simulink library "Library_SII"  (R2014b)
settings: Solver=ode45  StartTime=0.0  StopTime=10.0  RelTol=1e-3
libraries: fl_lib x77, Library_SII x44, nesl_utility x33, powerlib x15, mblibv1 x11, simulink x6, elec_lib x5, powerlib_extras x1
(part 1 of 4)
settings Model: Creator=Cedrick  LastModifiedBy=Cedrick

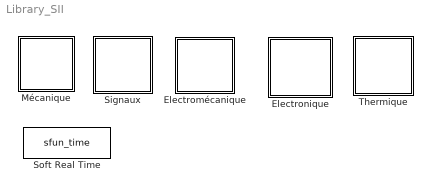
== system Library_SII ==
  Electromécanique : Subsystem
      mask Display: image(imread('Electromecanique.bmp'))
  Electronique : Subsystem
      mask Display: image(imread('Electronique.bmp'))
  Mécanique : Subsystem  mask(Mecanique){}
      mask Display: image(imread('Mecanique.bmp'))
  Signaux : Subsystem
      mask Display: image(imread('Signaux.bmp'))
  Soft Real Time : S-Function  FunctionName=sfun_time  Parameters=x  EnableBusSupport=off  mask{x=1}
      mask prompts: x "Time Scaling Factor"
      mask Display:
      | color('red')
      | disp('Soft Real Time')
  Thermique : Subsystem
      mask Display: image(imread('Thermique.bmp'))

== system Library_SII/Electromécanique ==
  Moteur CC (SPS-SM) : Subsystem  Tag=Moteur  Description=Moteur CC  mask(Moteur CC){axe=[1 0 0], R=0.989, L=0.0000718, K=1.39e-3, J=1.06e-6, kv=0.0002953, kc=0}
      mask prompts: axe "Vecteur directeur [x y z]"; R "Resistance (ohm)"; L "Inductance (H)"; K "Constante de vitesse (V/rpm)"; J "Inertie de l'arbre (kg.m^2)"; kv "Coefficient de frottement visqueux (N.m.s)"; kc "Coefficient de frottement sec"
      mask help:
      | Moteur à courant continu à aimants permanents.
      | L'axe du moteur est défini par le "Vecteur directeur"
      | et par la position du CS relié au stator.
      | Les autres paramètres sont fournis par les constructeurs de moteur.
      |
      | Les ports A+ et A- sont des ports physiques SimPowerSystems.
      | Les ports Stator et Rotor sont des ports mécaniques SimMechanics.
      mask Display:
      | image(imread('Motor.png'))
      | port_label('lconn', 1, 'Stator')
      | port_label('rconn', 1, 'Rotor')
      | port_label('lconn', 2, 'A+')
      | port_label('rconn', 2, 'A-')
  Moteur CC (SPS-SS) : Subsystem  Tag=Moteur  Description=Moteur CC  mask(Moteur CC){R=0.989, L=0.0000718, K=1.39e-3, J=1.06e-6, kv=0.0002953, kc=0}
      mask prompts: R "Resistance (ohm)"; L "Inductance (H)"; K "Constante de vitesse (V/rpm)"; J "Inertie de l'arbre (kg.m^2)"; kv "Coefficient de frottement visqueux (N.m.s)"; kc "Coefficient de frottement sec"
      mask help:
      | Moteur à courant continu à aimants permanents.
      | Les paramètres sont fournis par les constructeurs de moteur.
      |
      | Les ports A+ et A- sont des ports physiques SimPowerSystems.
      | Les ports Stator et Rotor sont des ports mécaniques SimScape.
      mask Display:
      | image(imread('Motor.png'))
      | port_label('lconn', 1, 'Stator')
      | port_label('rconn', 1, 'Rotor')
      | port_label('lconn', 2, 'A+')
      | port_label('rconn', 2, 'A-')
  Moteur PaP (SPS-SS) : Subsystem  Tag=Moteur  Description=Moteur PaP  mask(Moteur CC){R=0.989, L=0.0000718, K=1.39e-3, J=1.06e-6, kv=0.0002953, kc=0}
      mask prompts: R "Resistance (ohm)"; L "Inductance (H)"; K "Constante de vitesse (V/rpm)"; J "Inertie de l'arbre (kg.m^2)"; kv "Coefficient de frottement visqueux (N.m.s)"; kc "Coefficient de frottement sec"
      mask help:
      | Moteur à courant continu à aimants permanents.
      | Les paramètres sont fournis par les constructeurs de moteur.
      |
      | Les ports A+ et A- sont des ports physiques SimPowerSystems.
      | Les ports Stator et Rotor sont des ports mécaniques SimScape.
      mask Display:
      | image(imread('moteur_pap.jpg'))
      | port_label('lconn', 1, 'Stator')
      | port_label('rconn', 1, 'Rotor')
      | port_label('lconn', 2, 'A+')
      | port_label('rconn', 2, 'A-')
      | port_label('lconn', 3, 'B+')
      | port_label('rconn', 3, 'B-')

== system Library_SII/Electronique ==
  Ampèremètre : Subsystem  mask(Ampèremètre){}
      mask help: Ampèremètre avec un signal de sortie au format Simulink
      mask Display:
      | plot([184.371736831963;184.043550999396;183.062154110669;181.436997554304;179.183732476342;176.324059051243;172.885517497347;168.901222849516;164.409546043246;159.453744381582;154.081544943642;148.344684946756;142.298413488781;136.000959469086;129.512970812418;122.896930396238;116.216554306448;109.536178216657;102.920137800477;96.4321491438092;90.134695124114;84.0884236661391;78.3515636692533;72.979364231313;68.0235625696485;63.5318857633786;59.5475911155478;56.1090495616519;53.2493761365527;50.9961110585907;49.3709545022264;48.3895576134986;48.0613717809319;48.3895576134986;49.3709545022264;50.9961110585907;53.2493761365528;56.109049561652;59.547591115548;63.5318857633788;68.0235625696487;72.9793642313131;78.3515636692534;84.0884236661394;90.1346951241142;96.4321491438093;102.920137800477;109.536178216657;116.216554306448;122.896930396238;129.512970812418;136.000959469086;142.298413488781;148.344684946756;154.081544943642;159.453744381582;164.409546043246;168.901222849516;172.885517497347;176.324059051243;179.183732476342;181.436997554304;183.062154110669;184.043550999396;184.371736831963;184.371736831963], [130.389304831624;123.708928741834;117.092888325653;110.604899668986;104.307445649291;98.2611741913157;92.5243141944298;87.1521147564895;82.1963130948251;77.7046362885552;73.7203416407244;70.2818000868285;67.4221266617293;65.1688615837672;63.5437050274029;62.5623081386751;62.2341223061085;62.5623081386751;63.5437050274029;65.1688615837672;67.4221266617293;70.2818000868285;73.7203416407244;77.7046362885552;82.1963130948251;87.1521147564896;92.5243141944299;98.2611741913158;104.307445649291;110.604899668986;117.092888325653;123.708928741834;130.389304831624;137.069680921414;143.685721337595;150.173709994262;156.471164013958;162.517435471932;168.254295468818;173.626494906759;178.582296568423;183.073973374693;187.058268022524;190.49680957642;193.356483001519;195.609748079481;197.234904635845;198.216301524573;198.54448735714;198.216301524573;197.234904635845;195.609748079481;193.356483001519;190.49680957642;187.058268022524;183.073973374693;178.582296568423;173.626494906759;168.254295468818;162.517435471933;156.471164013958;150.173709994263;143.685721337595;137.069680921415;130.389304831624;130.389304831624])
      | plot([0;240.936758928001;240.936758928001;0;0], [255.109509453177;255.109509453177;0;0;255.109509453177])
      | plot([134.798604995012;113.382004201412], [102.043803781271;158.734805881977])
      | plot([113.696954213083;92.9102534428239], [158.419855870306;102.043803781271])
      | plot([143.617205321789;124.720204621553], [102.043803781271;102.043803781271])
      | plot([101.41390375793;84.406603127718], [102.043803781271;102.043803781271])
      | plot([99.2092536762357;127.554754726589], [119.051104411483;119.051104411483])
      | plot([48.1873517856002;0], [130.389304831624;130.389304831624])
      | plot([184.245756827295;212.591257877648;212.591257877648;240.936758928001], [130.389304831624;130.389304831624;65.194652415812;65.194652415812])
      | ;
      | color('red');
      | port_label('output', 1,'I')
      | port_label('LConn', 1,'+')
      | port_label('RConn', 1,'-')
  Cellule Photovoltaique SPS : Subsystem  mask(Cellule Photovoltaique SPS){Voc=0.6, Isc=5, Tjref=25, alpha=3.4e-4, TXI=3, EG=1.11, Rs=0.01, Rsh=50, Eref=1000, N=1.5}
      mask prompts: Voc "Tension à vide (V)"; Isc "Courant de court circuit (A)"; Tjref "Temperature de référence (°C)"; alpha "Coef de courant en température (°C^-1)"; TXI "Coef d'influence de la T°"; EG "Energie d'activation (eV)"; Rs "Résistance interne (Ohms)"; Rsh "Résistance de shunt (Ohm)"; Eref "Ensoleillement de référence (W/m²)"; N "Facteur de qualité"
      mask help:
      | Modèle d'une cellule photovoltaique.
      | En entrée :
      |   Ta : Température ambiante (°C)
      |   Ir : Irradiation (W/m²)
      |
      | En sortie :
      |   Ports physiques SimPowerSystems
      mask init:
      | % Charge de l'electron
      | q = 1.602e-19; % C
      | % Constante de Boltzmann
      | k = 1.38e-23;
      | % Degrés --> Kelvin
      | Kel = 273.15;
      | 
      | qkT = q/(k*(Tjref+Kel)); % 38.9358 à 25°C
      | 
      | % Courant de saturation de la diode (A)
      | % pour I = 0 (circuit ouvert)
      | I0d = ((Voc+Rs*Isc)/Rsh-Isc)/(exp(qkT*Rs*Isc/N)-exp(qkT*Voc/N));
      | 
      | % Courant de référence (A)
      | % pour U = 0 (court circuit)
      | I0 = Isc*(1+Rs/Rsh)+I0d*(exp(qkT*Rs*Isc/N)-1);
      | 
      | % Coef de tension en température (influe sur Iph)
      | beta = -2.17e-3; % mV/°C
      mask Display:
      | image(imread('cellulePV_poly.jpg'))
      | port_label('input', 1, 'Ta')
      | port_label('input', 2, 'Ir')
      | port_label('rconn', 1, '+')
      | port_label('rconn', 2, '-')
  Cellule Photovoltaique avec capteurs U et I SimElectronics : Subsystem  mask(Cellule Photovoltaique (SimElectronics)){typcell=polycristallin, Icc=4.5, Vco=0.601, Tcell=25, shunt=0, mesure=off, IRef=1000, TRef=25, Qf=1.4}
      mask prompts: typcell "Type"; Icc "Courant de court-circuit (A)"; Vco "Tension de circuit ouvert (V)"; Tcell "Température de cellule (°C)"; shunt "Shunter"; mesure "Mesurer le courant et la tension"; IRef "Irradiance de référence (W/m²)"; TRef "Température de référence (°C)"; Qf "Facteur de qualité"
      mask help:
      | Modèle d'une cellule photovoltaique.
      |  - mesure courant/tension
      |  - possibilité de shunter la cellule (par programmation)
      |
      | En entrée :
      |   Ir : Irradiation (W/m²)
      |
      | Connectique : ports physiques SimElectronics
      |
      | Caractéristiques :
      |     Courant de court-circuit (A)
      |     Tension de circuit ouvert (V)
      |     Température (°C) et irradiance (W/m²) de référence
      |
      | Température
      |     Température de cellule (°C)
      |
      | Il est possible de "tester" cette cellule grâce à l'interface graphique "CellulePV_IHM".
      |
      | Voir aussi la classe "pnl_etat_cellule.m" pour la programmation d'IHM.
      mask TypeOptions typcell: monocristallin | polycristallin | amorphe
      mask Callback typcell:
      | t = get_param(gcb, 'typcell');
      | switch t
      |     case 'monocristallin'
      |         n = '1.4';
      |     case 'polycristallin'
      |         n = '2';
      |     case 'amorphe'
      |         n = '10';
      | end
      | set_param(gcb, 'Qf', n)
      mask Display:
      | t = get_param(gcb, 'typcell');
      | switch t
      |     case 'monocristallin'
      |         image(imread('cellulePV_mono.jpg'))
      |     case 'polycristallin'
      |         image(imread('cellulePV_poly.jpg'))
      |     case 'amorphe'
      |         image(imread('cellulePV_amorphe.jpg'))
      | end
      | 
      | port_label('input', 1, 'Ir')
      | port_label('rconn', 1, '+')
      | port_label('rconn', 2, '-')
      | port_label('output', 1, 'I')
      | port_label('output', 2, 'U')
  Diode : Subsystem  mask(Diode){I0d=1e-6, N=1.5}
      mask prompts: I0d "Courant de saturation (A)"; N "Facteur de qualité"
      mask help:
      | Diode selon le modèle de Shockley :
      | Id = Is*(exp(Vd/(N*Vt))-1)
      |     avec Vt = k*Tj/q
      |
      |     Id : courant traversant la diode
      |     Vd : tension aux bornes de la diode
      |
      |     k : constante de Boltzmann
      |     q : charge de l'electron
      |
      | La température de jonction Tj (K) est donnée par le port Simulink Tj.
      |
      | Les paramètres intrinsèques à la diode sont :
      |     N : facteur de qualité (entre 1 et 2 pour les diodes en silicium)
      |     Id : courant de saturation de la diode (A)
      |
      | Les bornes A et C correspondent à l'anode et à la cathode de la diode.
      mask init:
      | % Charge de l'electron
      | q = 1.602e-19; % C
      | % Constante de Boltzmann
      | k = 1.38e-23;
      | % Degrés --> Kelvin
      | Kel = 273.15;
      | 
      | Tj = 300;
      mask Display:
      | image(imread('Diode.png'))
      | port_label('lconn', 1, 'A')
      | port_label('rconn', 1, 'C')
      | port_label('input', 1, 'Tj')
  Interrupteur : Subsystem  mask(Interrupteur){}
      mask help: Interrupteur avec signal de commutation au format Simulink
      mask Display:
      | patch([178.308949107304;178.270428219378;178.155236532808;177.964483406507;177.700005897356;177.364351068347;176.960751458971;176.493093954097;175.965882351142;175.384193986049;174.753630835755;174.080265568098;173.370583058705;172.631417938094;171.869888770445;171.093329497935;170.309218810871;169.525108123807;168.748548851298;167.987019683648;167.247854563037;166.538172053645;165.864806785988;165.234243635694;164.6525552706;164.125343667646;163.657686162771;163.254086553395;162.918431724386;162.653954215236;162.463201088934;162.348009402364;162.309488514438;162.348009402364;162.463201088934;162.653954215236;162.918431724386;163.254086553395;163.657686162771;164.125343667646;164.6525552706;165.234243635694;165.864806785988;166.538172053645;167.247854563037;167.987019683648;168.748548851298;169.525108123807;170.309218810871;171.093329497935;171.869888770445;172.631417938094;173.370583058705;174.080265568098;174.753630835754;175.384193986049;175.965882351142;176.493093954096;176.960751458971;177.364351068347;177.700005897356;177.964483406507;178.155236532808;178.270428219378;178.308949107304;178.308949107304], [113.618216710165;112.834106023101;112.057546750592;111.296017582942;110.556852462331;109.847169952939;109.173804685282;108.543241534988;107.961553169894;107.43434156694;106.966684062065;106.563084452689;106.22742962368;105.962952114529;105.772198988228;105.657007301658;105.618486413732;105.657007301658;105.772198988228;105.962952114529;106.22742962368;106.563084452689;106.966684062065;107.43434156694;107.961553169894;108.543241534988;109.173804685282;109.847169952939;110.556852462331;111.296017582942;112.057546750592;112.834106023101;113.618216710165;114.402327397229;115.178886669738;115.940415837388;116.679580957999;117.389263467392;118.062628735048;118.693191885343;119.274880250436;119.80209185339;120.269749358265;120.673348967641;121.00900379665;121.273481305801;121.464234432102;121.579426118672;121.617947006598;121.579426118672;121.464234432102;121.273481305801;121.00900379665;120.673348967641;120.269749358265;119.80209185339;119.274880250436;118.693191885343;118.062628735048;117.389263467392;116.679580957999;115.940415837388;115.178886669738;114.402327397229;113.618216710165;113.618216710165], [0;0;0])
      | plot([178.308949107304;178.270428219378;178.155236532808;177.964483406507;177.700005897356;177.364351068347;176.960751458971;176.493093954097;175.965882351142;175.384193986049;174.753630835755;174.080265568098;173.370583058705;172.631417938094;171.869888770445;171.093329497935;170.309218810871;169.525108123807;168.748548851298;167.987019683648;167.247854563037;166.538172053645;165.864806785988;165.234243635694;164.6525552706;164.125343667646;163.657686162771;163.254086553395;162.918431724386;162.653954215236;162.463201088934;162.348009402364;162.309488514438;162.348009402364;162.463201088934;162.653954215236;162.918431724386;163.254086553395;163.657686162771;164.125343667646;164.6525552706;165.234243635694;165.864806785988;166.538172053645;167.247854563037;167.987019683648;168.748548851298;169.525108123807;170.309218810871;171.093329497935;171.869888770445;172.631417938094;173.370583058705;174.080265568098;174.753630835754;175.384193986049;175.965882351142;176.493093954096;176.960751458971;177.364351068347;177.700005897356;177.964483406507;178.155236532808;178.270428219378;178.308949107304;178.308949107304], [113.618216710165;112.834106023101;112.057546750592;111.296017582942;110.556852462331;109.847169952939;109.173804685282;108.543241534988;107.961553169894;107.43434156694;106.966684062065;106.563084452689;106.22742962368;105.962952114529;105.772198988228;105.657007301658;105.618486413732;105.657007301658;105.772198988228;105.962952114529;106.22742962368;106.563084452689;106.966684062065;107.43434156694;107.961553169894;108.543241534988;109.173804685282;109.847169952939;110.556852462331;111.296017582942;112.057546750592;112.834106023101;113.618216710165;114.402327397229;115.178886669738;115.940415837388;116.679580957999;117.389263467392;118.062628735048;118.693191885343;119.274880250436;119.80209185339;120.269749358265;120.673348967641;121.00900379665;121.273481305801;121.464234432102;121.579426118672;121.617947006598;121.579426118672;121.464234432102;121.273481305801;121.00900379665;120.673348967641;120.269749358265;119.80209185339;119.274880250436;118.693191885343;118.062628735048;117.389263467392;116.679580957999;115.940415837388;115.178886669738;114.402327397229;113.618216710165;113.618216710165])
      | patch([64.926944905892;64.888424017966;64.7732323313963;64.5824792050947;64.3180016959439;63.9823468669351;63.5787472575591;63.1110897526843;62.5838781497303;62.0021897846366;61.3716266343423;60.6982613666856;59.988578857293;59.2494137366818;58.4878845690323;57.7113252965232;56.927214609459;56.1431039223949;55.3665446498857;54.6050154822362;53.8658503616251;53.1561678522324;52.4828025845758;51.8522394342815;51.2705510691878;50.7433394662337;50.275681961359;49.872082351983;49.5364275229742;49.2719500138234;49.0811968875218;48.9660052009521;48.9274843130261;48.9660052009521;49.0811968875218;49.2719500138234;49.5364275229742;49.8720823519831;50.275681961359;50.7433394662338;51.2705510691878;51.8522394342816;52.4828025845758;53.1561678522325;53.8658503616251;54.6050154822362;55.3665446498858;56.143103922395;56.927214609459;57.7113252965232;58.4878845690323;59.2494137366818;59.988578857293;60.6982613666856;61.3716266343422;62.0021897846366;62.5838781497303;63.1110897526843;63.5787472575591;63.982346866935;64.3180016959439;64.5824792050947;64.7732323313963;64.888424017966;64.926944905892;64.926944905892], [113.618216710165;112.834106023101;112.057546750592;111.296017582942;110.556852462331;109.847169952939;109.173804685282;108.543241534988;107.961553169894;107.43434156694;106.966684062065;106.563084452689;106.22742962368;105.962952114529;105.772198988228;105.657007301658;105.618486413732;105.657007301658;105.772198988228;105.962952114529;106.22742962368;106.563084452689;106.966684062065;107.43434156694;107.961553169894;108.543241534988;109.173804685282;109.847169952939;110.556852462331;111.296017582942;112.057546750592;112.834106023101;113.618216710165;114.402327397229;115.178886669738;115.940415837388;116.679580957999;117.389263467392;118.062628735048;118.693191885343;119.274880250436;119.80209185339;120.269749358265;120.673348967641;121.00900379665;121.273481305801;121.464234432102;121.579426118672;121.617947006598;121.579426118672;121.464234432102;121.273481305801;121.00900379665;120.673348967641;120.269749358265;119.80209185339;119.274880250436;118.693191885343;118.062628735048;117.389263467392;116.679580957999;115.940415837388;115.178886669738;114.402327397229;113.618216710165;113.618216710165], [0;0;0])
      | plot([64.926944905892;64.888424017966;64.7732323313963;64.5824792050947;64.3180016959439;63.9823468669351;63.5787472575591;63.1110897526843;62.5838781497303;62.0021897846366;61.3716266343423;60.6982613666856;59.988578857293;59.2494137366818;58.4878845690323;57.7113252965232;56.927214609459;56.1431039223949;55.3665446498857;54.6050154822362;53.8658503616251;53.1561678522324;52.4828025845758;51.8522394342815;51.2705510691878;50.7433394662337;50.275681961359;49.872082351983;49.5364275229742;49.2719500138234;49.0811968875218;48.9660052009521;48.9274843130261;48.9660052009521;49.0811968875218;49.2719500138234;49.5364275229742;49.8720823519831;50.275681961359;50.7433394662338;51.2705510691878;51.8522394342816;52.4828025845758;53.1561678522325;53.8658503616251;54.6050154822362;55.3665446498858;56.143103922395;56.927214609459;57.7113252965232;58.4878845690323;59.2494137366818;59.988578857293;60.6982613666856;61.3716266343422;62.0021897846366;62.5838781497303;63.1110897526843;63.5787472575591;63.982346866935;64.3180016959439;64.5824792050947;64.7732323313963;64.888424017966;64.926944905892;64.926944905892], [113.618216710165;112.834106023101;112.057546750592;111.296017582942;110.556852462331;109.847169952939;109.173804685282;108.543241534988;107.961553169894;107.43434156694;106.966684062065;106.563084452689;106.22742962368;105.962952114529;105.772198988228;105.657007301658;105.618486413732;105.657007301658;105.772198988228;105.962952114529;106.22742962368;106.563084452689;106.966684062065;107.43434156694;107.961553169894;108.543241534988;109.173804685282;109.847169952939;110.556852462331;111.296017582942;112.057546750592;112.834106023101;113.618216710165;114.402327397229;115.178886669738;115.940415837388;116.679580957999;117.389263467392;118.062628735048;118.693191885343;119.274880250436;119.80209185339;120.269749358265;120.673348967641;121.00900379665;121.273481305801;121.464234432102;121.579426118672;121.617947006598;121.579426118672;121.464234432102;121.273481305801;121.00900379665;120.673348967641;120.269749358265;119.80209185339;119.274880250436;118.693191885343;118.062628735048;117.389263467392;116.679580957999;115.940415837388;115.178886669738;114.402327397229;113.618216710165;113.618216710165])
      | plot([56.927214609459;161.805568495765], [113.618216710165;56.927214609459])
      | plot([227.000220911577;113.618216710165;113.618216710165], [170.309218810871;170.309218810871;82.4381655547768])
      | patch([0;227.23643342033;227.23643342033;0;0;0.472425017505884;0.472425017505884;226.764008402824;226.764008402824;0.472425017505884;0], [227.23643342033;227.23643342033;0;0;227.23643342033;226.764008402824;0.472425017505884;0.472425017505884;226.764008402824;226.764008402824;227.23643342033], [1;1;1])
      | plot([170.309218810871;198.654719861224;198.654719861224;227.000220911577], [113.618216710165;113.618216710165;56.927214609459;56.927214609459])
      | plot([56.927214609459;0.236212508752942], [113.618216710165;113.618216710165])
      | ;
      | color('red');
      | port_label('LConn', 1,'')
      | port_label('RConn', 1,'')
  Panneau photovoltaique SimElectronics : Subsystem  mask(Panneau Photovoltaïque (SimElectronics)){typcell=polycristallin, s=8, Icc=4.5, Vco=0.601, Tcell=30, C=[2.1         3.1         3.2], D=[0  50  50], shunt_diode=[1 1 1 1]}
      mask prompts: typcell "Type"; s "Nombre de cellules en série (x4)"; Icc "Courant de court-circuit (A)"; Vco "Tension de circuit ouvert (V)"; Tcell "Température de cellule (°C)"; C "Cellules occultées"; D "Degré d'occultation (%)"; shunt_diode "shunt diode"
      mask help:
      | Panneau Photovoltaïque 12V maxi
      |  - au maximum 4 rangées de 9 cellules occultables partiellement
      |  - possibilité de desactiver (shunter) les cellules par rangées de 4
      |  - possibilité d'utiliser ou non des diodes ByPass.
      |
      | Les caractéristiques Vco, et Icc des cellulles sont données pour les
      | valeurs de référence Tref = 25°C et Iref = 1000W/m².
      |
      | Entrées :
      |   Ir : Irradiance W/m²
      |
      | Sorties (3 vecteurs) :
      |   Ui : tensions aux bornes des cellules
      |   Ii : courants traversant les cellules
      |   Id : courants traversant les diodes de shunt
      |
      | Connectique : SimElectronics
      |
      | Pour gérer ce bloc, il est conseillé d'utiliser l'interface graphique "ModulePV_IHM.m".
      |
      | Voir aussi la classe "pnl_etat_module.m" pour la programmation d'IHM.
      mask init:
      | % Liste des valeurs degré d'occultation
      | % (1 pour toutes par défaut)
      | G = ones(4,9);
      | for l = 1:4
      |     for c = 1:9
      |         lc = l+c/10;
      |         G(l,c) = 1;
      |         for o = 1:length(C)
      |             if C(o) == lc
      |                 G(l,c) = D(o)/100;
      |             end
      |         end
      |     end
      | end
      | 
      | 
      | % Réalisation de la structure
      | for i = 1:9
      |     if i <= s
      |         v = '0';
      |     else
      |         v = '1';
      |     end
      |     for cell = 1:4
      |         ncell = [gcb, '/Cellule ', num2str(cell), '.', num2str(i)];
      |         set_param(ncell, 'shunt', v)
      |     end
      | end
      mask TypeOptions typcell: monocristallin | polycristallin | amorphe
      mask Callback typcell:
      | t = get_param(gcb, 'typcell');
      | c = find_system(gcb, 'Regexp', 'on', 'LookUnderMasks', 'all',...
      |     'FollowLinks', 'on', 'Name', 'Cellule+');
      | n = length(c);
      | for i = 1:n
      |     a = c{i,1};
      |     set_param(a, 'typcell', t )
      | end
      mask Callback D:
      | D = str2num(get_param(gcb, 'D'));
      | for d = 1:length(D)
      |     if D(d) > 100
      |         error('Le degré d''occultation doit être compris entre 0% et 100%')
      |     end
      | end
      mask Display:
      | image(imread('modulePV.png'))
      | port_label('input', 1, 'Ir')
      | port_label('rconn', 1, '+')
      | port_label('rconn', 2, '-')
      | port_label('output', 1, 'Ui')
      | port_label('output', 2, 'Ii')
      | port_label('output', 3, 'Id')
  Simscape<->SPS : Subsystem  mask(Convertisseur Simscape SimPowerSystems){}
      mask help:
      | Convertisseur Simscape SimPowerSystems
      |
      | Attention : à utiliser avec prudence : créé des "algebraic loops"
      | web([docroot '/toolbox/simulink/ug/f7-8243.html#f7-19688'])
  Voltmètre : Subsystem  mask(Voltmètre){}
      mask help: Voltmètre avec un signal de sortie au format Simulink
      mask Display:
      | plot([90.7056033611298;147.396605461836], [106.138153932989;127.554754726589])
      | plot([147.081655450165;90.7056033611298], [127.239804714918;148.026505485177])
      | plot([90.7056033611298;90.7056033611298], [97.3195536062121;116.216554306448])
      | plot([90.7056033611298;90.7056033611298], [139.522855170071;156.530155800283])
      | plot([184.371736831963;184.043550999396;183.062154110669;181.436997554304;179.183732476342;176.324059051243;172.885517497347;168.901222849516;164.409546043246;159.453744381582;154.081544943642;148.344684946756;142.298413488781;136.000959469086;129.512970812418;122.896930396238;116.216554306448;109.536178216657;102.920137800477;96.4321491438092;90.134695124114;84.0884236661391;78.3515636692533;72.979364231313;68.0235625696485;63.5318857633786;59.5475911155478;56.1090495616519;53.2493761365527;50.9961110585907;49.3709545022264;48.3895576134986;48.0613717809319;48.3895576134986;49.3709545022264;50.9961110585907;53.2493761365528;56.109049561652;59.547591115548;63.5318857633788;68.0235625696487;72.9793642313131;78.3515636692534;84.0884236661394;90.1346951241142;96.4321491438093;102.920137800477;109.536178216657;116.216554306448;122.896930396238;129.512970812418;136.000959469086;142.298413488781;148.344684946756;154.081544943642;159.453744381582;164.409546043246;168.901222849516;172.885517497347;176.324059051243;179.183732476342;181.436997554304;183.062154110669;184.043550999396;184.371736831963;184.371736831963], [130.389304831624;123.708928741834;117.092888325653;110.604899668986;104.307445649291;98.2611741913157;92.5243141944298;87.1521147564895;82.1963130948251;77.7046362885552;73.7203416407244;70.2818000868285;67.4221266617293;65.1688615837672;63.5437050274029;62.5623081386751;62.2341223061085;62.5623081386751;63.5437050274029;65.1688615837672;67.4221266617293;70.2818000868285;73.7203416407244;77.7046362885552;82.1963130948251;87.1521147564896;92.5243141944299;98.2611741913158;104.307445649291;110.604899668986;117.092888325653;123.708928741834;130.389304831624;137.069680921414;143.685721337595;150.173709994262;156.471164013958;162.517435471932;168.254295468818;173.626494906759;178.582296568423;183.073973374693;187.058268022524;190.49680957642;193.356483001519;195.609748079481;197.234904635845;198.216301524573;198.54448735714;198.216301524573;197.234904635845;195.609748079481;193.356483001519;190.49680957642;187.058268022524;183.073973374693;178.582296568423;173.626494906759;168.254295468818;162.517435471933;156.471164013958;150.173709994263;143.685721337595;137.069680921415;130.389304831624;130.389304831624])
      | plot([0;240.936758928001;240.936758928001;0;0], [255.109509453177;255.109509453177;0;0;255.109509453177])
      | plot([48.1873517856002;0], [130.389304831624;130.389304831624])
      | plot([184.245756827295;212.591257877648;212.591257877648;240.936758928001], [130.389304831624;130.389304831624;62.3601023107767;62.3601023107767])
      | ;
      | color('red');
      | port_label('output', 1,'V')
      | port_label('LConn', 1,'+')
      | port_label('RConn', 1,'-')

== system Library_SII/Mécanique ==
  Capteur de puissance mécanique de rotation : Subsystem  mask(Capteur de puissance mécanique de rotation){}
      mask help:
      | Le bloc représente un capteur de puissance mécanique de rotation.
      | R et C sont des ports physiques conservatifs.
      |
      | P, T et W sont des ports Simulink délivrant les valeurs de :
      |  - la puissance mécanique traversant le bloc (en W)
      |  - le couple transmis à travers le bloc (en Nm)
      |  - la vitesse de rotation (en rad/s)
      |
      | Ces valeurs sont calculées par rapport au référentiel Ref.
      mask Display:
      | plot([149.600878633536;150.016472378793;150.47508104106;150.972287968219;151.50330478576;152.063017511447;152.646035805762;153.246744883819;153.859359588817;154.477980106257;155.096648782383;155.709407499646;156.310355056631;156.893703999851;157.453836360095;157.985357756531;158.483149347555;158.942417128023;159.358738098149;159.728102859405;160.046954227227;160.312221488639;160.521349974904;160.672325664379;160.763694578642;160.794576785101;160.764674871227;160.674276808796;160.524253180566;160.316048796087;160.051668777399;159.733659248606;159.365082815313;158.949489070056;158.490880407788;157.993673480629;157.462656663088;156.908284800231], [156.971389291536;157.430657072004;157.84697804213;158.216342803387;158.535194171208;158.80046143262;159.009589918885;159.16056560836;159.251934522623;159.282816729083;159.252914815208;159.162516752777;159.012493124547;158.804288740068;158.53990872138;158.221899192587;157.853322759294;157.437729014037;156.979120351769;156.48191342461;155.950896607069;155.391183881382;154.808165587067;154.20745650901;153.594841804012;152.976221286573;152.357552610446;151.744793893183;151.143846336199;150.560497392978;150.000365032735;149.468843636298;148.971052045274;148.511784264806;148.095463294681;147.726098533424;147.407247165603;147.144199990631])
      | plot([152.057635404444;152.93604260309;153.834625296826;154.744729643097;155.657590839533;156.564417533794;157.45647648909;158.325176690034;159.162152078811;159.959342124889;160.709069452336;161.404113777147;162.037781442523;162.603969882449;163.097226392739;163.512800643557;163.846690427691;164.095680203997;164.257372064819;164.330208829146;164.313489039122;164.27939575172], [142.228020686971;141.979030910664;141.817339049842;141.744502285515;141.761222075539;141.867337399197;142.061826307913;142.342815767178;142.707599694895;143.152665022428;143.673725527376;144.265763112236;144.923076131425;145.639334301243;146.40763966397;147.220593018964;148.070365181011;148.948772379657;149.847355073393;150.757459419663;151.6703206161;152.055850472277])
      | %plot([116.468514315784;116.438789536125;116.349901463023;116.202706137216;115.998621130155;115.739611892022;115.42817282337;115.067303252679;114.660478551187;114.211616663162;113.725040373958;113.205435679231;112.657806656235;112.087427271827;111.499790591278;110.900555877058;110.29549408704;109.690432297022;109.091197582803;108.503560902254;107.933181517846;107.38555249485;106.865947800123;106.379371510919;105.930509622894;105.523684921402;105.162815350711;104.851376282059;104.592367043926;104.388282036865;104.241086711057;104.152198637956;104.122473858297;104.152198637956;104.241086711057;104.388282036865;104.592367043926;104.851376282059;105.162815350711;105.523684921402;105.930509622894;106.379371510919;106.865947800123;107.38555249485;107.933181517846;108.503560902254;109.091197582803;109.690432297022;110.29549408704;110.900555877058;111.499790591278;112.087427271827;112.657806656235;113.205435679231;113.725040373958;114.211616663162;114.660478551187;115.067303252679;115.42817282337;115.739611892022;115.998621130155;116.202706137216;116.349901463023;116.438789536125;116.468514315784;116.468514315784], [111.618284136057;111.013222346039;110.413987631819;109.826350951271;109.255971566862;108.708342543866;108.188737849139;107.702161559936;107.253299671911;106.846474970419;106.485605399728;106.174166331075;105.915157092943;105.711072085881;105.563876760074;105.474988686973;105.445263907313;105.474988686973;105.563876760074;105.711072085881;105.915157092943;106.174166331075;106.485605399728;106.846474970419;107.253299671911;107.702161559936;108.188737849139;108.708342543866;109.255971566862;109.826350951271;110.413987631819;111.013222346039;111.618284136057;112.223345926075;112.822580640295;113.410217320843;113.980596705252;114.528225728247;115.047830422975;115.534406712178;115.983268600203;116.390093301695;116.750962872386;117.062401941038;117.321411179171;117.525496186232;117.67269151204;117.761579585141;117.7913043648;117.761579585141;117.67269151204;117.525496186232;117.321411179171;117.062401941038;116.750962872386;116.390093301695;115.983268600203;115.534406712178;115.047830422975;114.528225728247;113.980596705252;113.410217320843;112.822580640295;112.223345926075;111.618284136057;111.618284136057])
      | plot([239.23602886498;238.828071429858;237.608127977604;235.587947230552;232.78698463364;229.232214987837;224.957872668068;220.005121927465;214.421660463109;208.261260061133;201.583248745024;194.451939414329;186.936010476274;179.107844435155;171.042830809261;162.818640088593;154.514475725591;146.210311362589;137.986120641921;129.921107016027;122.092940974909;114.577012036853;107.445702706158;100.76769139005;94.607290988073;89.0238295237172;84.0710787831142;79.7967364633452;76.2419668175427;73.4410042206305;71.4208234735788;70.2008800213248;69.7929225862026;70.2008800213248;71.4208234735788;73.4410042206306;76.2419668175428;79.7967364633454;84.0710787831144;89.0238295237174;94.6072909880733;100.76769139005;107.445702706159;114.577012036853;122.092940974909;129.921107016027;137.986120641921;146.210311362589;154.514475725591;162.818640088593;171.042830809261;179.107844435155;186.936010476274;194.451939414329;201.583248745024;208.261260061133;214.421660463109;220.005121927465;224.957872668068;229.232214987837;232.78698463364;235.587947230552;237.608127977604;238.828071429858;239.23602886498;239.23602886498], [155.774275772274;147.47628550917;139.258209428443;131.199192095207;123.376846251889;115.866505365088;108.740498123116;102.067451871182;95.9116316925529;90.3323215006612;85.3832531026163;81.1120887325275;77.5599620381344;74.7610819412943;72.742403187363;71.5233667562631;71.1157126352191;71.5233667562631;72.742403187363;74.7610819412943;77.5599620381345;81.1120887325275;85.3832531026164;90.3323215006612;95.9116316925529;102.067451871182;108.740498123116;115.866505365089;123.376846251889;131.199192095207;139.258209428443;147.47628550917;155.774275772274;164.072266035377;172.290342116104;180.34935944934;188.171705292658;195.682046179459;202.808053421432;209.481099673365;215.636919851994;221.216230043886;226.165298441931;230.43646281202;233.988589506413;236.787469603253;238.806148357184;240.025184788284;240.432838909328;240.025184788284;238.806148357184;236.787469603253;233.988589506413;230.43646281202;226.165298441931;221.216230043886;215.636919851994;209.481099673365;202.808053421432;195.682046179459;188.171705292658;180.34935944934;172.290342116105;164.072266035378;155.774275772274;155.774275772274])
      | plot([252.715889364481;252.243022716633;250.828976737403;248.487369462568;245.240751850236;241.120390602797;236.165967051481;230.425195003451;223.953361231755;216.812793033479;209.072257983804;200.806301666664;192.094529760025;183.020841389688;173.672621134841;164.139897466795;154.514475725591;144.889053984387;135.356330316341;126.008110061494;116.934421691157;108.222649784518;99.9566934673787;92.2161584177032;85.075590219427;78.6037564477313;72.8629843997015;67.9085608483856;63.7881996009461;60.5415819886144;58.199974713779;56.7859287345493;56.3130620867014;56.7859287345493;58.1999747137791;60.5415819886146;63.7881996009463;67.9085608483858;72.8629843997018;78.6037564477315;85.0755902194273;92.2161584177035;99.9566934673791;108.222649784519;116.934421691157;126.008110061494;135.356330316341;144.889053984387;154.514475725591;164.139897466796;173.672621134841;183.020841389688;192.094529760025;200.806301666664;209.072257983803;216.812793033479;223.953361231755;230.425195003451;236.165967051481;241.120390602797;245.240751850236;248.487369462568;250.828976737403;252.243022716633;252.715889364481;252.715889364481], [154.514475725591;144.895228084285;135.36861905618;126.026395093992;116.958526921455;108.252343066071;99.9916888376535;92.2561188521535;85.1201308772245;78.6524483779929;72.9153586725213;67.9641130708855;63.8463947748555;60.6018596625959;58.2617543808809;56.8486154228053;56.3760520890355;56.8486154228053;58.2617543808809;60.6018596625959;63.8463947748555;67.9641130708856;72.9153586725213;78.652448377993;85.1201308772246;92.2561188521536;99.9916888376536;108.252343066072;116.958526921455;126.026395093992;135.36861905618;144.895228084285;154.514475725591;164.133723366898;173.660332395002;183.002556357191;192.070424529728;200.776608385111;209.037262613529;216.772832599029;223.908820573958;230.37650307319;236.113592778661;241.064838380297;245.182556676327;248.427091788587;250.767197070302;252.180336028377;252.652899362147;252.180336028377;250.767197070301;248.427091788587;245.182556676327;241.064838380297;236.113592778661;230.37650307319;223.908820573958;216.772832599029;209.037262613529;200.776608385111;192.070424529728;183.002556357191;173.660332395002;164.133723366898;154.514475725592;154.514475725591])
      | plot([154.514475725591;129.948374815285;179.017586633563;154.514475725591], [240.369848906994;203.583687543869;203.583687543869;240.369848906994])
      | %plot([105.382273904979;149.60125554353], [115.271704271436;156.971085816622])
      | plot([144.688035361469;144.688035361469], [152.057865634561;203.583687543869])
      | plot([164.277926087379;164.277926087379], [152.057865634561;203.583687543869])
      | plot([159.112745895982;159.616665914655], [149.60125554353;149.60125554353])
      | %plot([115.208714269102;159.364705905318], [107.901873998344;149.60125554353])
      | plot([0;311.800511553884;311.800511553884;0;0], [311.800511553884;311.800511553884;0;0;311.800511553884])
      | ;
      | color('red');
      | port_label('LConn', 1,'R')
      | port_label('RConn', 1,'C')
      | port_label('LConn', 2,'Ref')
      | port_label('output', 1,'P')
      | port_label('output', 2,'T')
      | port_label('output', 3,'W')
      | %port_label('RConn', 3,'A')
  Embrayage SM : Subsystem  mask(Embrayage){axe=[0 0 1]}
      mask prompts: axe "Axe de la  liaison [x y z]"
      mask help:
      | Embrayage, basé sur une liaison pivot.
      |   C = Signal Simulink de commande
      |     C > 0 : état embrayé (transmission intégralle de la puissance)
      |     C = 0 : état débrayé (équivalent à une liaison pivot)
      |
      | Indiquer l'axe de la liaison par ses composantes dans World.
      mask Display:
      | image(imread('Mécanique/embrayage.png'))
      | port_label('lconn', 1, 'B')
      | port_label('rconn', 1, 'F')
      | port_label('input', 1, 'C')
  Engrenage droit SS : Subsystem  mask(Réducteur à engrenages droit){r=2, n=0.8, J=0.001}
      mask prompts: r "Rapport de transmission"; n "Rendement"; J "Inertie (kg/m^2)"
      mask help:
      | Réducteur à engrenages droit
      | P = Pignon
      | R = Roue
      | Ref = Référence
      |
      | Le rapport de réduction est défini par : wp/wr
      | Le rendement doit être compris entre 0.1 et 1
      mask Callback n:
      | ren = str2num(get_param(gcb,'n'));
      | if or((ren < 0.1),(ren > 1));
      |     errordlg('Le rendement doit etre compris entre 0.1 et 1','Erreur');
      | end;
      mask Display:
      | plot([0] , [0]);
      | 
      | color('red');
      | plot([30, 100] , [150, 150]);
      | plot([90, 110] , [180, 180]);
      | plot([90, 110] , [120, 120]);
      | plot([100, 100] , [120, 180]);
      | 
      | color('blue');
      | plot([100, 180] , [50, 50]);
      | plot([100, 100] , [0, 120]);
      | plot([90, 110] , [0, 0]);
      | 
      | color('black');
      | %image(imread('RoueVisSSFin.jpg'))
      | port_label('lconn', 1, 'P');
      | port_label('lconn', 2, 'Ref');
      | port_label('rconn', 1, 'R');
  Roue - Vis sans fin SS : Subsystem  mask(Engrenage à Roue et Vis sans fin){r=5, f=0.15, J=0.01, B=60}
      mask prompts: r "Rapport de transmission"; f "Coefficient de frottement"; J "Inertie (kg/m^2)"; B "Angle de denture  de la roue (°)"
      mask help:
      | Engrenage à Roue et Vis sans fin :
      | R = Roue
      | V = Vis
      | Ref = Référence
      |
      | Le rapport de transmission est défini par : r = Wv/Wr
      |
      | Les valeurs de l'angle de denture de la roue
      | et du coefficient de frottement
      | permettent de calculer le rendement (voir l'aide pour plus d'informations)
      | Selon que la vis ou la roue soit motrice, ce rendement varie
      | et l'on peut avoir irréversibilité.
      mask init:
      | % Angle de frottement (en rad)
      | P = atan(f);
      | 
      | % Angle de denture (en rad)
      | Br = pi*B/180;
      | 
      | % Rendements selon le sens
      | n1 = tan(Br)/tan(Br+P);
      | n2 = tan(Br-P)/tan(Br);
      mask Help:
      | Le rendement est calculé, selon le sens, par les expressions :
      |  - Vis motrice : n1 = tan(B)/tan(B+P)
      |  - Roue motrice : n2 = tan(B-P)/tan(B)
      | 
      | avec P = atan(f) : Angle de frottement
      mask Callback B:
      | if ( str2num(get_param(gcb, 'B')) <= 0);
      |      errordlg('L''angle de denture ne peut pas être négatif !','Erreur');
      | end;
      mask Display:
      | image(imread('Mécanique/RoueVisSSFin.jpg'));
      | port_label('lconn', 1, 'V');
      | port_label('lconn', 2, 'Ref');
      | port_label('rconn', 1, 'R');
  Roue libre SM : Subsystem  mask(Roue libre){axe=[1 0 0], kv=0.01}
      mask prompts: axe "Vecteur directeur [x y z]"; kv "Coefficient de frottement visqueux (Nm/(rad/s))"
      mask help:
      | Roue libre, basée sur une liaison pivot, mais la rotation n'est possible
      | que dans un seul sens.
      | Pour inverser le sens, inverser les connections B et F.
      |
      | Indiquer l'axe de la liaison par ses composantes dans World.
      mask Display:
      | image(imread('Mécanique/Roue_libre.png'))
      | port_label('lconn', 1, 'B')
      | port_label('rconn', 1, 'F')

== system Library_SII/Signaux ==
  Contrôle de régime : Subsystem  mask(Controleur de régime){vl=0.8, al=1}
      mask prompts: vl "Vitesse limite (1/s)"; al "Accélération limite (1/s²)"
      mask help:
      | Permet de limiter la vitesse et l'accélération de variation d'un signal
      | à partir d'un échelon.
      mask Callback al:
      | if str2num(get_param(gcb, 'vl'))<=0
      | 	error('La vitesse limite doit être strictement positive !')
      | end
      | if str2num(get_param(gcb, 'al'))<=0
      | 	error('L''accélération limite doit être strictement positive')
      | end
      mask Display:
      | color('red');
      | x = [10 15 20 25 30 35 40 45 55 60 65 70 75 80 85 90];
      | y = [10 10.68 12.72 16.12 20.88 27 34.48 41.96 58.04 65.52 73 79.12 83.88 87.28 89.32 90];
      | plot(x/100, y/100);
      | plot(x/100, (y-1)/100);
      | plot(x/100, (y+1)/100);
  Frequence-Metre : Subsystem  mask(Fréquence-mètre){Ts=100e-6, Fs=6, spec=on, plage=[-1 -1]}
      mask prompts: Ts "Pèriode d'échantillonage (s)"; Fs "Fréquence de mesure (Hz)"; spec "Tracer un spectrogramme"; plage "Plage de fréquence du spectrogramme (-1 = auto)"
      mask help:
      | Estimation de la fréquence principale d'un signal.
      | - Période d'echantillonage : période en secondes entre deux échantillons
      | du signal. Le solveur doit être réglé en mode "Fixed-step" et cette période
      | doit être égale au paramètre "Fixed-step size".
      |
      | - Fréquence de mesure : fréquence entre deux mesures du fréquence-mètre en Hertz.
      |
      | La mesure est soumise à un compromis temps de calcul/précision.
      | Pour augmenter la précision, diminuer la période d'échantillonage
      | et choisir une fréquence de mesure au moins 10 fois inférieure à la fréquence
      | à mesurer.
      |
      | Pour afficher un spectrogramme, cocher la case "Tracer un spectrogramme"
      | et renseigner la plage de fréquence ([-1 -1] = auto)
      mask init:
      | N=fix((1/Fs)/Ts);
      mask Callback spec:
      | dd = get_param(gcb,'spec');
      | if strcmp(dd,'on'),
      |     set_param(gcb,'MaskEnables',{'on';'on';'on';'on'}),
      | else
      |     set_param(gcb,'MaskEnables',{'on';'on';'on';'off'}),
      | end
  Générateur de signal carré : Subsystem  mask(Générateur de signal carré){t=16, a=1, d=5}
      mask prompts: t "Retard (s)"; a "Amplitude"; d "Durée (s)"
      mask help:
      | Signal "carré" unique, à amplitude, durée et retard contrôlés.
      | Paramètres :
      |   Retard (s)
      |   Amplitude
      |   Durée (s)
      mask Display:
      | %origine
      | ox = 10;
      | oy = 10;
      | 
      | %fleche
      | l = 10;
      | e = 5;
      | 
      | %dimension
      | x = 300;
      | y = 200;
      | 
      | % ecarts
      | dx = 30;
      | dy = 30;
      | 
      | h = y-4*l;
      | 
      | %axes
      | color('black');
      | plot([dx;dx;x], [y;dy;dy])
      | plot([dx-e;dx;dx+e], [y-2*e;y;y-2*e])
      | plot([x-l;x;x-l], [dy-e;dy;dy+e])
      | plot([0], [0])
      | 
      | %textes
      | text(x/3,15, 't0')
      | text(dx,15, '0')
      | text(15,h, 'a')
      | text(x/2,h/2, 'd')
      | 
      | %courbe
      | color('red');
      | plot([dx;x/3;x/3;2*x/3;2*x/3;x-2*l], [dy; dy;h;h;dy;dy])
  Générateur de signal pas : Subsystem  mask(Générateur de signal carré){t=0.5, a=10, p=5}
      mask prompts: t "Retard (s)"; a "Amplitude"; p "Pente"
      mask help:
      | Signal "carré" unique, à amplitude, durée et retard contrôlés.
      | Paramètres :
      |   Retard (s)
      |   Amplitude
      |   Durée (s)
      mask Display:
      | %origine
      | ox = 10;
      | oy = 10;
      | 
      | %fleche
      | l = 10;
      | e = 5;
      | 
      | %dimension
      | x = 300;
      | y = 200;
      | 
      | % ecarts
      | dx = 30;
      | dy = 30;
      | 
      | h = y-4*l;
      | 
      | %axes
      | color('black');
      | plot([dx;dx;x], [y;dy;dy])
      | plot([dx-e;dx;dx+e], [y-2*e;y;y-2*e])
      | plot([x-l;x;x-l], [dy-e;dy;dy+e])
      | plot([0], [0])
      | 
      | %textes
      | text(x/3,15, 't0')
      | text(dx,15, '0')
      | text(15,h, 'a')
      | text(x/2,h/2, 'p')
      | 
      | %courbe
      | color('red');
      | plot([dx; x/3; 2*x/3; x-2*l], [dy; dy; h; h])
      | 
      | %image(imread('carre.jpg'))
  Trapèze : Subsystem  mask{a=1, t0=0, p=0.2, th=4}
      mask prompts: a "Amplitude"; t0 "Instant début (s)"; p "Pente"; th "Temps haut (s)"
      mask Display:
      | %origine
      | ox = 10;
      | oy = 10;
      | 
      | %fleche
      | l = 10;
      | e = 5;
      | 
      | %dimension
      | x = 300;
      | y = 200;
      | 
      | % ecarts
      | dx = 30;
      | dy = 30;
      | 
      | h = y-4*l;
      | 
      | %axes
      | color('black');
      | plot([dx;dx;x], [y;dy;dy])
      | plot([dx-e;dx;dx+e], [y-2*e;y;y-2*e])
      | plot([x-l;x;x-l], [dy-e;dy;dy+e])
      | plot([0], [0])
      | 
      | %textes
      | text(x/3,15, 't0')
      | text(dx,15, '0')
      | text(15,h, 'a')
      | text(x/2,h/2, 'p')
      | 
      | %courbe
      | color('red');
      | plot([dx; x/5; 2*x/5; 3*x/5; 4*x/5; x-2*l], [dy; dy; h; h; dy; dy])
      | 
      | 
      | %image(imread('carre.jpg'))
